simulink model "velo_pi"  (R2015a)
settings: Solver=ode3  StartTime=0.0  StopTime=10.0  FixedStep=ts  RelTol=1e-3
values from neighbouring files (symbols this model uses):
  K = 1.904071    [verify_parameter.m]
  T = 0.166667    [verify_parameter.m]
  u_offset = 1.5    [verify_parameter.m]
undefined symbols (not defined in the file or in its folder): Ki, Kp
libraries: arduinolib x2
settings Model: SimulationMode=external  ExtModeTrigDuration=2  Creator=shohei  LastModifiedBy=shohei
settings OptimizationCC: OptimizeModelRefInitCode=on  LifeSpan=1
settings DebuggingCC: UnderspecifiedInitializationDetection=Classic  MergeDetectMultiDrivingBlocksExec=none
settings HardwareCC: ProdBitPerInt=16  ProdBitPerPointer=8  ProdIntDivRoundTo=Zero  ProdEndianess=LittleEndian  ProdWordSize=8  ProdHWDeviceType=Atmel->AVR
settings RTWCC: SystemTargetFile=realtime.tlc  GenerateMakefile=off  TemplateMakefile=realtime.tmf  Description=Run on Target Hardware  RTWVerbose=off
settings ERTTargetCC: CombineOutputUpdateFcns=off  ExtModeTransport=3  ExtModeMexFile=ext_serial_win32_comm_rtt  ExtModeMexArgs=0 1 9600  ERTSrcFileBannerTemplate=realtime_code_template.cgt  ERTHdrFileBannerTemplate=realtime_code_template.cgt  ERTDataSrcFileTemplate=realtime_code_template.cgt  ERTDataHdrFileTemplate=realtime_code_template.cgt  ERTCustomFileTemplate=realtime_file_process.tlc

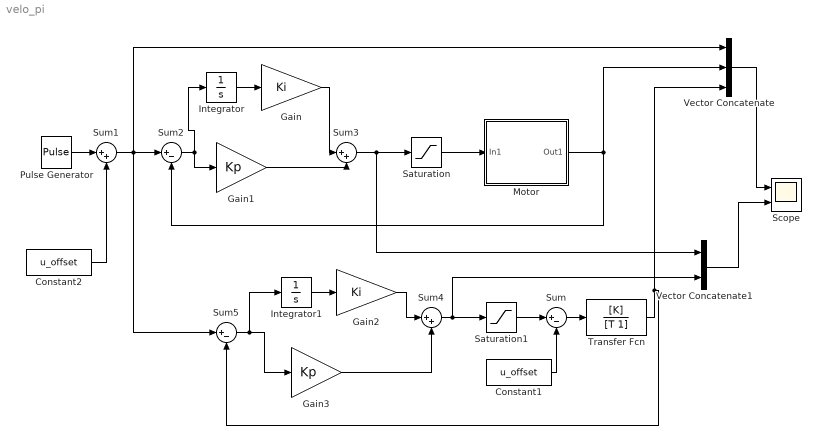
== system velo_pi ==
  Constant1 : Constant  Value=u_offset
  Constant2 : Constant  Value=u_offset
  Gain : Gain  Gain=Ki
  Gain1 : Gain  Gain=Kp
  Gain2 : Gain  Gain=Ki
  Gain3 : Gain  Gain=Kp
  Integrator : Integrator
  Integrator1 : Integrator
  "Motor " : Subsystem
  Pulse Generator : DiscretePulseGenerator  PulseType=Time based  Amplitude=3  PulseWidth=50  PhaseDelay=1
  Saturation : Saturate  UpperLimit=5  LowerLimit=0
  Saturation1 : Saturate  UpperLimit=5  LowerLimit=0
  Scope : Scope  NumInputPorts=2
      settings: YMin=-5~-5  YMax=5~5
  Sum : Sum  Inputs=|+-
  Sum1 : Sum  Inputs=|++
  Sum2 : Sum  Inputs=|+-
  Sum3 : Sum  Inputs=|++
  Sum4 : Sum  Inputs=|++
  Sum5 : Sum  Inputs=|+-
  Transfer Fcn : TransferFcn  Numerator=[K]  Denominator=[T 1]
  Vector Concatenate : Concatenate  NumInputs=3
  Vector Concatenate1 : Concatenate
  wires:
  Sum/1 -> Transfer Fcn/1
  Constant1/1 -> Sum/2
  "Motor "/1(Out1) -> Sum2/2, Vector Concatenate/2
  Vector Concatenate/1 -> Scope/1
  Integrator/1 -> Gain/1
  Sum2/1 -> Gain1/1, Integrator/1
  Gain/1 -> Sum3/1
  Gain1/1 -> Sum3/2
  Sum3/1 -> Saturation/1, Vector Concatenate1/1
  Sum5/1 -> Integrator1/1, Gain3/1
  Integrator1/1 -> Gain2/1
  Gain2/1 -> Sum4/1
  Gain3/1 -> Sum4/2
  Transfer Fcn/1 -> Sum5/2, Vector Concatenate/3
  Sum4/1 -> Saturation1/1, Vector Concatenate1/2
  Vector Concatenate1/1 -> Scope/2
  Saturation/1 -> "Motor "/1(In1)
  Saturation1/1 -> Sum/1
  Pulse Generator/1 -> Sum1/1
  Constant2/1 -> Sum1/2
  Sum1/1 -> Sum5/1, Vector Concatenate/1, Sum2/1

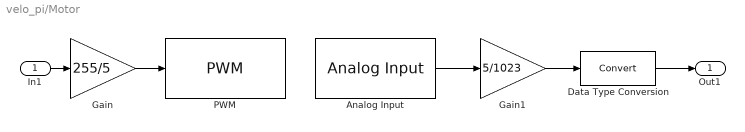
== system velo_pi/Motor  ==
  In1 : Inport
  Analog Input : arduinolib/Analog Input  pinNumber=5  sampleTime=ts  blockPlatform=arduino
  Data Type Conversion : DataTypeConversion
  Gain : Gain  Gain=255/5
  Gain1 : Gain  Gain=5/1023
  PWM : arduinolib/PWM  pinNumber=9  blockPlatform=arduino
  Out1 : Outport
  wires:
  Gain1/1 -> Data Type Conversion/1
  Gain/1 -> PWM/1
  Analog Input/1 -> Gain1/1
  In1/1 -> Gain/1
  Data Type Conversion/1 -> Out1/1
